simulink model "Phase3"  (R2016b)
settings: Solver=VariableStepAuto  StartTime=0.0  StopTime=40  RelTol=1e-3  EnableMultiTasking=on
settings Model: Creator=m.soleimani  LastModifiedBy=Sare
settings OptimizationCC: LifeSpan=inf
settings DebuggingCC: SFUnexpectedBacktrackingDiag=warning  SFNoUnconditionalDefaultTransitionDiag=warning  SFExecutionAtInitializationDiag=none
settings GRTTargetCC: TargetLangStandard=C89/C90 (ANSI)  GeneratePreprocessorConditionals=Disable all
settings ConfigComp: CovMetricSettings=dw  CovHtmlReporting=on  CovSaveCumulativeToWorkspaceVar=on  CovSaveSingleToWorkspaceVar=on  CovExternalEMLEnable=off

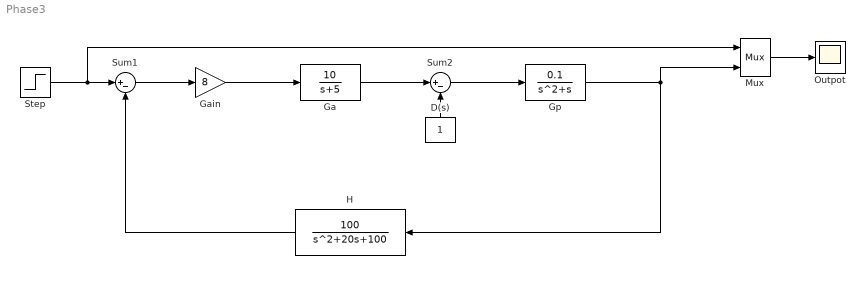
== system Phase3 ==
  " D(s)  " : Constant
  Ga : TransferFcn  Numerator=[10]  Denominator=[1 5]
  Gain : Gain  Gain=8
  Gp : TransferFcn  Numerator=[0.1]  Denominator=[1 1 0 ]
  H : TransferFcn  Numerator=[100]  Denominator=[1 20 100 ]
  Mux : Mux  Inputs=2
  Outpot : Scope
  Step : Step  After=4  SampleTime=0
  Sum1 : Sum  Inputs=|+-
  Sum2 : Sum  Inputs=|+-
  wires:
  H/1 -> Sum1/2
  Step/1 -> Mux/1, Sum1/1
  Mux/1 -> Outpot/1
  Gp/1 -> H/1, Mux/2
  Sum1/1 -> Gain/1
  " D(s)  "/1 -> Sum2/2
  Sum2/1 -> Gp/1
  Gain/1 -> Ga/1
  Ga/1 -> Sum2/1
